simulink model "rosslerSystemOriginal"  (R2018b)
settings: Solver=ode4  StartTime=0  StopTime=100  FixedStep=1e-3  RelTol=1e-3
settings Model: Creator=plazas  LastModifiedBy=Daples

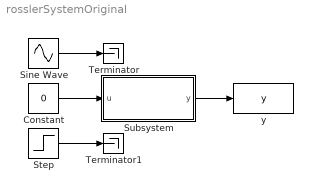
== system rosslerSystemOriginal ==
  "Constant " : Constant  Value=0
  "Sine Wave " : Sin  Amplitude=500  Bias=500  Frequency=5  SampleTime=0
  "Step " : Step  Time=40  After=1000  SampleTime=0
  Subsystem : Subsystem  mask{Ra=500, Rb=7500, Rc=17.5439, RCs=1, ci=[0 -6.78 0.02]}
      mask prompts: Ra "Resistance a"; Rb "Resistance b"; Rc "Resistance c"; RCs "Time speed (RC)"; ci "Initial Conditions"
      mask init:
      | x10 = ci(1);
      | x20 = ci(2);
      | y0 = ci(3);
      mask Display: disp("Rössler Attractor")
  Terminator : Terminator
  Terminator1 : Terminator
  y : ToWorkspace  VariableName=y  SampleTime=-1
  wires:
  Subsystem/1("y ") -> y/1
  "Constant "/1 -> Subsystem/1(u)
  "Sine Wave "/1 -> Terminator/1
  "Step "/1 -> Terminator1/1

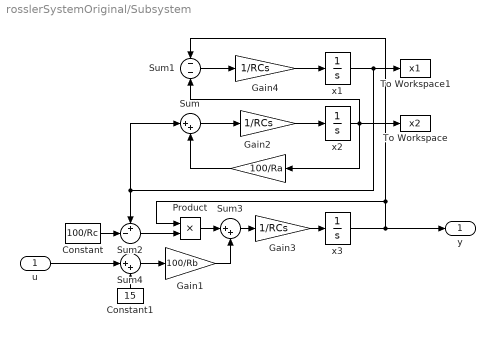
== system rosslerSystemOriginal/Subsystem ==
  u : Inport
  " " : Gain  Gain=1/RCs
  Constant : Constant  Value=100/Rc
  Constant1 : Constant  Value=15
  Gain1 : Gain  Gain=100/Rb
  Gain2 : Gain  Gain=100/Ra
  Gain3 : Gain  Gain=1/RCs
  Gain4 : Gain  Gain=1/RCs
  Product : Product
  Sum : Sum  Inputs=|++
  Sum1 : Sum  Inputs=--
  Sum2 : Sum  Inputs=+-|
  Sum3 : Sum  Inputs=|++
  Sum4 : Sum  Inputs=|++
  To Workspace : ToWorkspace  VariableName=x2  SampleTime=-1
  To Workspace1 : ToWorkspace  VariableName=x1  SampleTime=-1
  x1 : Integrator  InitialCondition=x10
  x2 : Integrator  InitialCondition=x20  AbsoluteTolerance=0
  "x3 " : Integrator  InitialCondition=y0
  "y " : Outport
  wires:
  Sum1/1 -> Gain4/1
  Gain2/1 -> Sum/2
  Sum2/1 -> Product/2
  Product/1 -> Sum3/1
  "x3 "/1 -> "y "/1, Sum1/1, Product/1
  x1/1 -> To Workspace1/1, Sum2/1, Sum/1
  Sum/1 -> " "/1
  Sum3/1 -> Gain3/1
  Constant/1 -> Sum2/2
  x2/1 -> Sum1/2, To Workspace/1, Gain2/1
  u/1 -> Sum4/1
  " "/1 -> x2/1
  Gain3/1 -> "x3 "/1
  Gain4/1 -> x1/1
  Gain1/1 -> Sum3/2
  Constant1/1 -> Sum4/2
  Sum4/1 -> Gain1/1
